simulink model "HW1"  (R2018a)
settings: Solver=VariableStepAuto  StartTime=0.0  StopTime=60  RelTol=1e-3
settings Model: Creator=User  LastModifiedBy=User

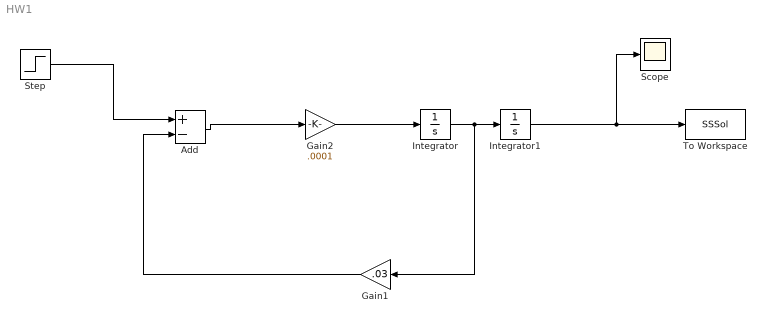
== system HW1 ==
  Add : Sum  Inputs=+-
  Gain1 : Gain  Gain=.03
  Gain2 : Gain  Gain=.0001
  Integrator : Integrator
  Integrator1 : Integrator
  Scope : Scope
  Step : Step  After=5  SampleTime=0
  To Workspace : ToWorkspace  VariableName=SSSol  SaveFormat=Timeseries  SampleTime=-1
  wires:
  Step/1 -> Add/1
  Gain2/1 -> Integrator/1
  Add/1 -> Gain2/1
  Integrator/1 -> Gain1/1, Integrator1/1
  Integrator1/1 -> Scope/1, To Workspace/1
  Gain1/1 -> Add/2
